simulink model "sm"  (R2025b)
settings: Solver=FixedStepAuto  StartTime=0.0  StopTime=10.0  RelTol=1e-3
model workspace (MAT data in the model file):
  SL_Bus_ROSEnable64bitIntegers = 1
undefined symbols (not defined in the file or in its folder): twist
libraries: ros2lib x5
settings Model: Creator=HP  LastModifiedBy=HP
settings OptimizationCC: DefaultParameterBehavior=Inlined  EnhancedBackFolding=on  PassReuseOutputArgsAs=Individual arguments  ZeroExternalMemoryAtStartup=off  ZeroInternalMemoryAtStartup=off  MaxStackSize=64  OptimizeBlockOrder=speed  DifferentSizesBufferReuse=on  OptimizationCustomize=off  EfficientTunableParamExpr=on
settings DebuggingCC: ParameterTunabilityLossMsg=error
settings SFSimCC: MATLABDynamicMemAlloc=off
settings RTWCC: SystemTargetFile=ert.tlc  HardwareBoard=Robot Operating System 2 (ROS 2)  TLCOptions="-aInlineSetEventsForThisBaseRateFcn=TLC_FALSE -aSuppressMultiTaskScheduler=TLC_FALSE  -aRateBasedStepFcn=0"  TemplateMakefile=ert_default_tmf  Toolchain=Colcon Tools  TargetLang=C++  Description=Embedded Coder
settings CodeAppCC: ForceParamTrailComments=on  IgnoreCustomStorageClasses=off  OperatorAnnotations=on  SimulinkDataObjDesc=on  SFDataObjDesc=on  InsertBlockDesc=on
settings ERTTargetCC: ExtModeTransport=2.0  ExtModeStaticAlloc=on  ExtModeMexFile=ext_xcp  ExtModeIntrfLevel=Level2 - Open  RootIOFormat=Structure reference  CodeInterfacePackaging=C++ class

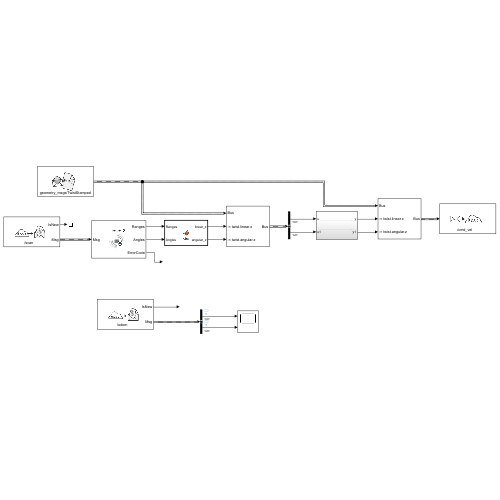
[thumbnail: Simulink's stored preview of the top-level diagram]
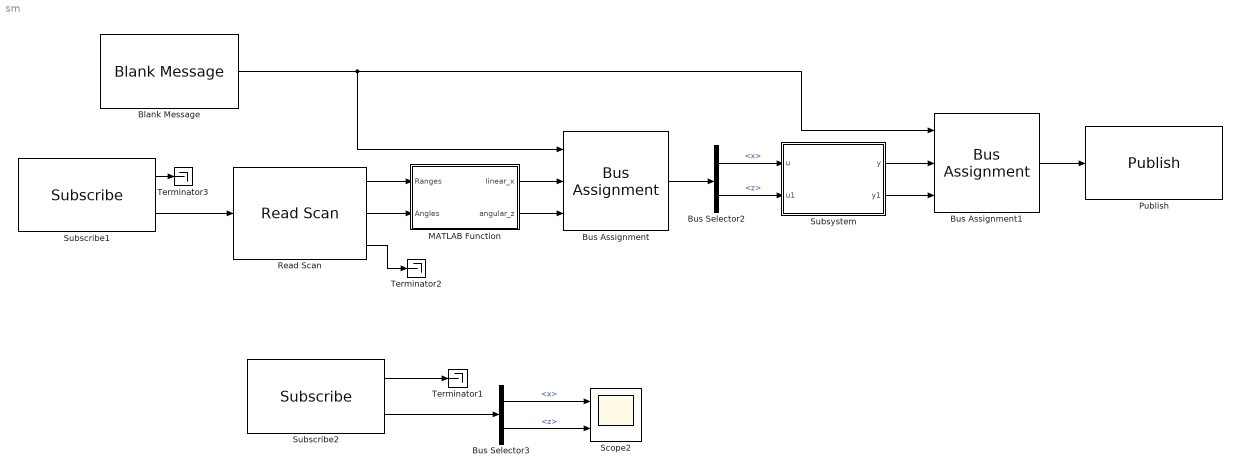
== system sm ==
  Blank Message : ros2lib/Blank Message  messageClass=Message  entityType=geometry_msgs/TwistStamped  messageType=geometry_msgs/TwistStamped  SampleTime=inf
  Bus Assignment : BusAssignment  AssignedSignals=twist.linear.x,twist.angular.z
  Bus Assignment1 : BusAssignment  AssignedSignals=twist.linear.x,twist.angular.z
  Bus Selector2 : BusSelector  OutputSignals=twist.linear.x,twist.angular.z
  Bus Selector3 : BusSelector  OutputSignals=twist.twist.linear.x,twist.twist.angular.z
  MATLAB Function : MATLAB Function  TreatAsAtomicUnit=on
  Publish : ros2lib/Publish  topicSource=Select from ROS network  topic=/cmd_vel  messageType=geometry_msgs/TwistStamped  QOSHistory=Keep last  QOSDepth=1  QOSReliability=Reliable  QOSDurability=Volatile  QOSDeadline=Inf  QOSLifespan=Inf  QOSLiveliness=Automatic  QOSLeaseDuration=Inf  QOSAvoidROSNamespaceConventions=off
  Read Scan : ros2lib/Read Scan  MaximumArrayLength=360  ShowAnglesOutput=on  ShowIntensityOutput=off  ShowErrorCodeOutput=on  VariableSizeOutputs=off
  Scope2 : Scope  NumInputPorts=2
      settings: ActiveDisplayYMinimum=-0.16061100000059383  ActiveDisplayYMaximum=0.084968400000077188  DataLoggingVariableName=PID2
  Subscribe1 : ros2lib/Subscribe  topicSource=Select from ROS network  topic=/scan  messageType=sensor_msgs/LaserScan  sampleTime=1  QOSHistory=Keep last  QOSDepth=1  QOSReliability=Reliable  QOSDurability=Volatile  QOSDeadline=Inf  QOSLifespan=Inf  QOSLiveliness=Automatic  QOSLeaseDuration=Inf  QOSAvoidROSNamespaceConventions=off
  Subscribe2 : ros2lib/Subscribe  topicSource=Select from ROS network  topic=/odom  messageType=nav_msgs/Odometry  sampleTime=-1  QOSHistory=Keep last  QOSDepth=1  QOSReliability=Reliable  QOSDurability=Volatile  QOSDeadline=Inf  QOSLifespan=Inf  QOSLiveliness=Automatic  QOSLeaseDuration=Inf  QOSAvoidROSNamespaceConventions=off
  Subsystem : Subsystem
  Terminator1 : Terminator
  Terminator2 : Terminator
  Terminator3 : Terminator
  wires:
  Bus Selector3/1 -> Scope2/1  "<x>"
  Subscribe2/1 -> Terminator1/1
  Blank Message/1 -> Bus Assignment/1, Bus Assignment1/1
  MATLAB Function/1(linear_x) -> Bus Assignment/2
  Bus Selector2/1 -> Subsystem/1(u)  "<x>"
  Subscribe2/2 -> Bus Selector3/1
  Bus Selector3/2 -> Scope2/2  "<z>"
  Bus Assignment1/1 -> Publish/1
  Bus Assignment/1 -> Bus Selector2/1
  MATLAB Function/2(angular_z) -> Bus Assignment/3
  Subscribe1/2 -> Read Scan/1
  Read Scan/2 -> MATLAB Function/2(Angles)
  Read Scan/1 -> MATLAB Function/1(Ranges)
  Read Scan/3 -> Terminator2/1
  Subscribe1/1 -> Terminator3/1
  Subsystem/2(y1) -> Bus Assignment1/3
  Subsystem/1(y) -> Bus Assignment1/2
  Bus Selector2/2 -> Subsystem/2(u1)  "<z>"

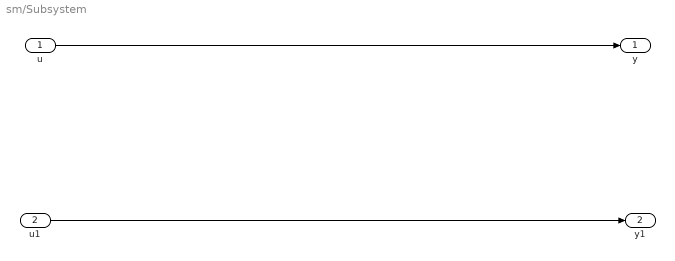
== system sm/Subsystem ==
  u : Inport
  u1 : Inport  Port=2
  y : Outport
  y1 : Outport  Port=2
  wires:
  u/1 -> y/1
  u1/1 -> y1/1

== matlab function sm/MATLAB Function ==
  data: Ranges input; linear_x output; Angles input; angular_z output
function [linear_x,angular_z] = stra(Ranges,Angles)
    linear_x = 0.1;
    angular_z = 0.1;
end
